simulink model "gm_parallel_delay_compensation_6phase"  (R2022a)
settings: Solver=FixedStepDiscrete  StartTime=0.0  StopTime=10.0  RelTol=1e-3
undefined symbols (not defined in the file or in its folder): f_c, L_d, L_q, L_x, L_y, p, psi_pm, R_ph
libraries: hdlmdlgenlib x10
settings Model: Creator=Andre Merx  LastModifiedBy=Andre Merx
settings SolverCC: AlgebraicLoopSolver=TrustRegion
settings DataIOCC: LimitDataPoints=on  SaveOutput=off  SaveTime=off
settings OptimizationCC: BlockReduction=off  ConditionallyExecuteInputs=off  DefaultParameterBehavior=Inlined  LifeSpan=inf
settings DebuggingCC: AlgebraicLoopMsg=error  InheritedTsInSrcMsg=none  SingleTaskRateTransMsg=error  UnconnectedInputMsg=warning  UnconnectedOutputMsg=warning  UnconnectedLineMsg=warning  AllowSymbolicDim=off  StrictBusMsg=ErrorOnBusTreatedAsVector  SFUnexpectedBacktrackingDiag=warning  SFNoUnconditionalDefaultTransitionDiag=warning  SFExecutionAtInitializationDiag=none  SFMachineParentedDataDiag=warning  ArithmeticOperatorsInVariantConditions=warning
settings HardwareCC: ProdBitPerPointer=32  ProdBitPerSizeT=32  ProdBitPerPtrDiffT=32  ProdLargestAtomicFloat=None  ProdIntDivRoundTo=Undefined  ProdEndianess=Unspecified  ProdWordSize=32  ProdHWDeviceType=ASIC/FPGA->ASIC/FPGA  ProdEqTarget=off
settings SFSimCC: SimUseLocalCustomCode=off  CustomCodeUndefinedFunction=UseInterfaceOnly
settings RTWCC: RTWUseLocalCustomCode=off
settings CodeAppCC: StateflowObjectComments=on
settings GRTTargetCC: TargetLangStandard=C89/C90 (ANSI)
settings ConfigComp: CovScope=ReferencedModels  CovMetricSettings=dw  CovSaveCumulativeToWorkspaceVar=on  CovSaveSingleToWorkspaceVar=on  CovExternalEMLEnable=off  CovSFcnEnable=off

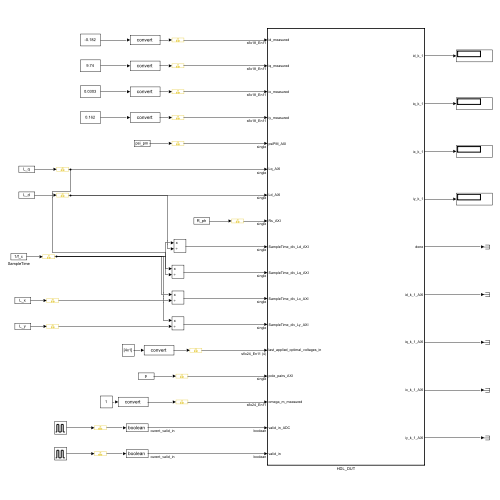
[thumbnail: Simulink's stored preview of the top-level diagram]
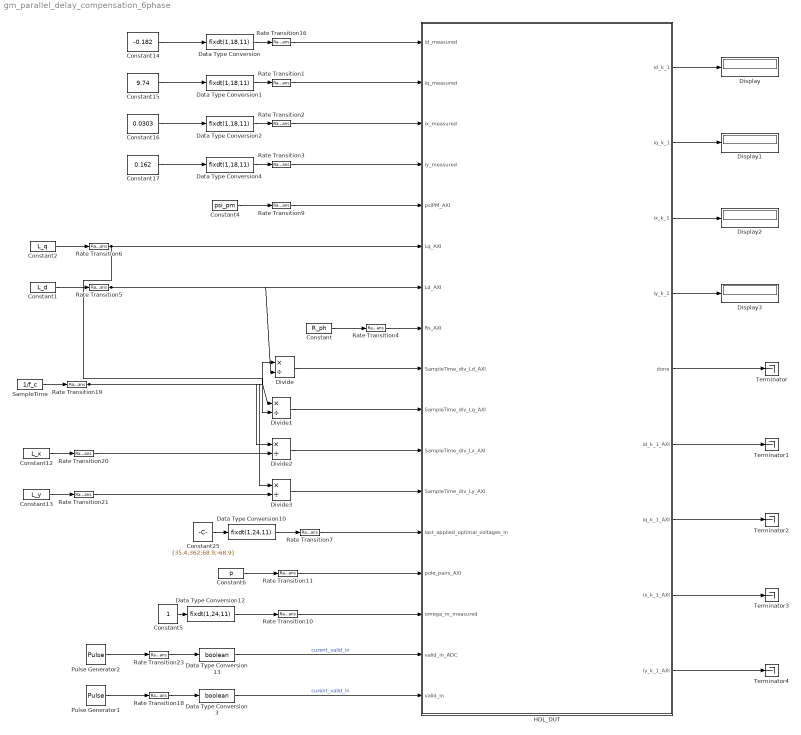
== system gm_parallel_delay_compensation_6phase ==
  Constant : Constant  Value=R_ph  OutDataTypeStr=single  SampleTime=-1
  Constant1 : Constant  Value=L_d  OutDataTypeStr=single  SampleTime=-1
  Constant12 : Constant  Value=L_x  OutDataTypeStr=single  SampleTime=-1
  Constant13 : Constant  Value=L_y  OutDataTypeStr=single  SampleTime=-1
  Constant14 : Constant  Value=-0.182
  Constant15 : Constant  Value=9.74
  Constant16 : Constant  Value=0.0303
  Constant17 : Constant  Value=0.162
  Constant2 : Constant  Value=L_q  OutDataTypeStr=single  SampleTime=-1
  Constant25 : Constant  Value=[35.4;362;68.9;-68.9]
  Constant4 : Constant  Value=psi_pm  OutDataTypeStr=single  SampleTime=-1
  Constant5 : Constant
  Constant6 : Constant  Value=p  OutDataTypeStr=single  SampleTime=-1
  Data Type Conversion{,1..2,4} (4 alike) : DataTypeConversion  OutDataTypeStr=fixdt(1,18,11)  SaturateOnIntegerOverflow=off  RndMeth=Floor
  Data Type Conversion10 : DataTypeConversion  OutDataTypeStr=fixdt(1,24,11)  SaturateOnIntegerOverflow=off  RndMeth=Floor
  Data Type Conversion12 : DataTypeConversion  OutDataTypeStr=fixdt(1,24,11)  SaturateOnIntegerOverflow=off  RndMeth=Floor
  Data Type Conversion13 : DataTypeConversion  OutDataTypeStr=boolean  SaturateOnIntegerOverflow=off  RndMeth=Floor
  Data Type Conversion3 : DataTypeConversion  OutDataTypeStr=boolean  SaturateOnIntegerOverflow=off  RndMeth=Floor
  Display{,1..3} (4 alike) : Display
  Divide{,1..3} (4 alike) : Product  Inputs=*/  RndMeth=Zero  SaturateOnIntegerOverflow=on
  HDL_DUT : Subsystem  TreatAsAtomicUnit=on
  Pulse Generator1 : DiscretePulseGenerator  PulseType=Time based  Period=1/f_c
  Pulse Generator2 : DiscretePulseGenerator  PulseType=Time based  Period=1/f_c
  Rate Transition{1..7,9..11,16,18..21,23} (16 alike) : RateTransition  OutPortSampleTime=Rt
  SampleTime : Constant  Value=1/f_c  OutDataTypeStr=single  SampleTime=-1
  Terminator{,1..4} (5 alike) : Terminator
  wires:
  Rate Transition7/1 -> HDL_DUT/13(last_applied_optimal_voltages_in)
  Data Type Conversion13/1 -> HDL_DUT/16(valid_in_ADC)  "curent_valid_in"
  Rate Transition23/1 -> Data Type Conversion13/1
  Pulse Generator2/1 -> Rate Transition23/1
  HDL_DUT/9(iy_k_1_AXI) -> Terminator4/1
  HDL_DUT/8(ix_k_1_AXI) -> Terminator3/1
  HDL_DUT/7(iq_k_1_AXI) -> Terminator2/1
  HDL_DUT/6(id_k_1_AXI) -> Terminator1/1
  Data Type Conversion10/1 -> Rate Transition7/1
  HDL_DUT/5(done) -> Terminator/1
  HDL_DUT/4(iy_k_1) -> Display3/1
  HDL_DUT/3(ix_k_1) -> Display2/1
  HDL_DUT/2(iq_k_1) -> Display1/1
  HDL_DUT/1(id_k_1) -> Display/1
  Constant17/1 -> Data Type Conversion4/1
  Rate Transition16/1 -> HDL_DUT/1(id_measured)
  Constant15/1 -> Data Type Conversion1/1
  Rate Transition1/1 -> HDL_DUT/2(iq_measured)
  Data Type Conversion4/1 -> Rate Transition3/1
  Rate Transition4/1 -> HDL_DUT/8(Rs_AXI)
  Rate Transition5/1 -> Divide/2, HDL_DUT/7(Ld_AXI)
  Constant6/1 -> Rate Transition11/1
  Constant16/1 -> Data Type Conversion2/1
  Data Type Conversion/1 -> Rate Transition16/1
  Constant4/1 -> Rate Transition9/1
  Data Type Conversion2/1 -> Rate Transition2/1
  Data Type Conversion1/1 -> Rate Transition1/1
  Constant14/1 -> Data Type Conversion/1
  Rate Transition3/1 -> HDL_DUT/4(iy_measured)
  Rate Transition2/1 -> HDL_DUT/3(ix_measured)
  Rate Transition10/1 -> HDL_DUT/15(omega_m_measured)
  Rate Transition9/1 -> HDL_DUT/5(psiPM_AXI)
  Constant5/1 -> Data Type Conversion12/1
  Data Type Conversion12/1 -> Rate Transition10/1
  Constant/1 -> Rate Transition4/1
  Rate Transition6/1 -> Divide1/2, HDL_DUT/6(Lq_AXI)
  Constant1/1 -> Rate Transition5/1
  Constant2/1 -> Rate Transition6/1
  Data Type Conversion3/1 -> HDL_DUT/17(valid_in)  "curent_valid_in"
  Pulse Generator1/1 -> Rate Transition18/1
  Constant12/1 -> Rate Transition20/1
  Constant13/1 -> Rate Transition21/1
  Rate Transition19/1 -> Divide2/1, Divide3/1, Divide1/1, Divide/1
  Divide1/1 -> HDL_DUT/10(SampleTime_div_Lq_AXI)
  Rate Transition11/1 -> HDL_DUT/14(pole_pairs_AXI)
  Rate Transition20/1 -> Divide2/2
  Divide3/1 -> HDL_DUT/12(SampleTime_div_Ly_AXI)
  Rate Transition18/1 -> Data Type Conversion3/1
  Rate Transition21/1 -> Divide3/2
  Divide2/1 -> HDL_DUT/11(SampleTime_div_Lx_AXI)
  SampleTime/1 -> Rate Transition19/1
  Divide/1 -> HDL_DUT/9(SampleTime_div_Ld_AXI)
  Constant25/1 -> Data Type Conversion10/1

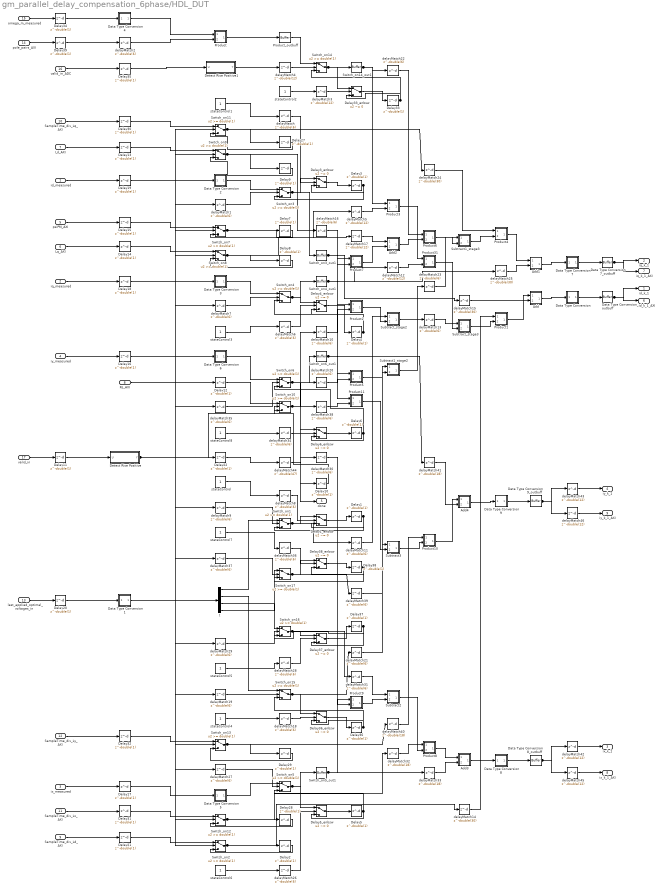
== system gm_parallel_delay_compensation_6phase/HDL_DUT ==
  id_measured : Inport  OutDataTypeStr=fixdt(1, 18, 11)  PortDimensions=1  SampleTime=1e-08
  iq_measured : Inport  Port=2  OutDataTypeStr=fixdt(1, 18, 11)  PortDimensions=1  SampleTime=1e-08
  ix_measured : Inport  Port=3  OutDataTypeStr=fixdt(1, 18, 11)  PortDimensions=1  SampleTime=1e-08
  iy_measured : Inport  Port=4  OutDataTypeStr=fixdt(1, 18, 11)  PortDimensions=1  SampleTime=1e-08
  psiPM_AXI : Inport  Port=5  OutDataTypeStr=single  PortDimensions=1  SampleTime=1e-08
  Lq_AXI : Inport  Port=6  OutDataTypeStr=single  PortDimensions=1  SampleTime=1e-08
  Ld_AXI : Inport  Port=7  OutDataTypeStr=single  PortDimensions=1  SampleTime=1e-08
  Rs_AXI : Inport  Port=8  OutDataTypeStr=single  PortDimensions=1  SampleTime=1e-08
  SampleTime_div_Ld_AXI : Inport  Port=9  OutDataTypeStr=single  PortDimensions=1  SampleTime=1e-08
  SampleTime_div_Lq_AXI : Inport  Port=10  OutDataTypeStr=single  PortDimensions=1  SampleTime=1e-08
  SampleTime_div_Lx_AXI : Inport  Port=11  OutDataTypeStr=single  PortDimensions=1  SampleTime=1e-08
  SampleTime_div_Ly_AXI : Inport  Port=12  OutDataTypeStr=single  PortDimensions=1  SampleTime=1e-08
  last_applied_optimal_voltages_in : Inport  Port=13  OutDataTypeStr=fixdt(1, 24, 11)  PortDimensions=[4]  SampleTime=1e-08
  pole_pairs_AXI : Inport  Port=14  OutDataTypeStr=single  PortDimensions=1  SampleTime=1e-08
  omega_m_measured : Inport  Port=15  OutDataTypeStr=fixdt(1, 24, 11)  PortDimensions=1  SampleTime=1e-08
  valid_in_ADC : Inport  Port=16  OutDataTypeStr=boolean  PortDimensions=1  SampleTime=1e-08
  valid_in : Inport  Port=17  OutDataTypeStr=boolean  PortDimensions=1  SampleTime=1e-08
  Add : Subsystem
      mask Display: disp('NFP\nadd');
  Add1 : Subsystem
      mask Display: disp('NFP\nadd');
  Add2 : Subsystem
      mask Display: disp('NFP\nadd');
  Add3 : Subsystem
      mask Display: disp('NFP\nadd');
  Add4 : Subsystem
      mask Display: disp('NFP\nadd');
  Data Type Conversion : Subsystem
      mask Display: disp('NFP\nconv');
  Data Type Conversion1 : Subsystem
      mask Display: disp('NFP\nconv');
  Data Type Conversion2 : Subsystem
      mask Display: disp('NFP\nconv');
  Data Type Conversion3 : Subsystem
      mask Display: disp('NFP\nconv');
  Data Type Conversion4 : Subsystem
      mask Display: disp('NFP\nconv');
  Data Type Conversion5 : Subsystem
      mask Display: disp('NFP\nconv');
  Data Type Conversion6 : Subsystem
      mask Display: disp('NFP\nconv');
  Data Type Conversion7 : Subsystem
      mask Display: disp('NFP\nconv');
  Data Type Conversion7_outbuff : hdlmdlgenlib/Buffer
      settings: SourceProductBaseCode=SL
  Data Type Conversion8 : Subsystem
      mask Display: disp('NFP\nconv');
  Data Type Conversion8_outbuff : hdlmdlgenlib/Buffer
      settings: SourceProductBaseCode=SL
  Data Type Conversion9 : Subsystem
      mask Display: disp('NFP\nconv');
  Data Type Conversion9_outbuff : hdlmdlgenlib/Buffer
      settings: SourceProductBaseCode=SL
  Data Type Conversion_outbuff : hdlmdlgenlib/Buffer
      settings: SourceProductBaseCode=SL
  Delay{1..22,27..39} (35 alike) : Delay  DelayLength=double(1)  InitialCondition=0  SampleTime=1e-08
  Delay1_enbsw : Switch  Criteria=u2 ~= 0  Threshold=double(0)  OutDataTypeStr=single  SampleTime=1e-08  SaturateOnIntegerOverflow=off  InputSameDT=off
  Delay33_enbsw : Switch  Criteria=u2 ~= 0  Threshold=double(0)  OutDataTypeStr=single  SampleTime=1e-08  SaturateOnIntegerOverflow=off  InputSameDT=off
  Delay36_enbsw : Switch  Criteria=u2 ~= 0  Threshold=double(0)  OutDataTypeStr=single  SampleTime=1e-08  SaturateOnIntegerOverflow=off  InputSameDT=off
  Delay37_enbsw : Switch  Criteria=u2 ~= 0  Threshold=double(0)  OutDataTypeStr=single  SampleTime=1e-08  SaturateOnIntegerOverflow=off  InputSameDT=off
  Delay38_enbsw : Switch  Criteria=u2 ~= 0  Threshold=double(0)  OutDataTypeStr=single  SampleTime=1e-08  SaturateOnIntegerOverflow=off  InputSameDT=off
  Delay3_enbsw : Switch  Criteria=u2 ~= 0  Threshold=double(0)  OutDataTypeStr=single  SampleTime=1e-08  SaturateOnIntegerOverflow=off  InputSameDT=off
  Delay4_enbsw : Switch  Criteria=u2 ~= 0  Threshold=double(0)  OutDataTypeStr=single  SampleTime=1e-08  SaturateOnIntegerOverflow=off  InputSameDT=off
  Delay5_enbsw : Switch  Criteria=u2 ~= 0  Threshold=double(0)  OutDataTypeStr=single  SampleTime=1e-08  SaturateOnIntegerOverflow=off  InputSameDT=off
  Delay6_enbsw : Switch  Criteria=u2 ~= 0  Threshold=double(0)  OutDataTypeStr=single  SampleTime=1e-08  SaturateOnIntegerOverflow=off  InputSameDT=off
  Detect Rise Positive : Subsystem  mask(Detect Rise Positive){vinit=double(0), InputProcessing=Elements as channels (sample based), OutDataTypeStr=boolean}
      mask prompts: vinit "Simulink:masks:InitialCondition_MP"; InputProcessing "Simulink:masks:InputProcessing_MP"; OutDataTypeStr "Simulink:masks:OutputDataType_MP"
      mask help: Simulink:masks:DetectRisePositive_MD
      mask init:
      | InputProcessing = 'Elements as channels (sample based)';
      | OutDataTypeStr = 'boolean';
      | vinit = double(0);
      mask TypeOptions InputProcessing: Simulink:masks:ColumnsAsChannelsFrameBased | Simulink:masks:ElementsAsChannelsSampleBased
      mask TypeOptions OutDataTypeStr: Simulink:masks:uint8 | Simulink:masks:boolean
      mask Display: fprintf('U > 0\n&  NOT\nU/z > 0')
  Detect Rise Positive1 : Subsystem  mask(Detect Rise Positive){vinit=double(0), InputProcessing=Elements as channels (sample based), OutDataTypeStr=boolean}
      mask prompts: vinit "Simulink:masks:InitialCondition_MP"; InputProcessing "Simulink:masks:InputProcessing_MP"; OutDataTypeStr "Simulink:masks:OutputDataType_MP"
      mask help: Simulink:masks:DetectRisePositive_MD
      mask init:
      | InputProcessing = 'Elements as channels (sample based)';
      | OutDataTypeStr = 'boolean';
      | vinit = double(0);
      mask TypeOptions InputProcessing: Simulink:masks:ColumnsAsChannelsFrameBased | Simulink:masks:ElementsAsChannelsSampleBased
      mask TypeOptions OutDataTypeStr: Simulink:masks:uint8 | Simulink:masks:boolean
      mask Display: fprintf('U > 0\n&  NOT\nU/z > 0')
  Product : Subsystem
      mask Display: disp('NFP\nmul');
  Product1 : Subsystem
      mask Display: disp('NFP\nmul');
  Product10 : Subsystem
      mask Display: disp('NFP\nmul');
  Product11 : Subsystem
      mask Display: disp('NFP\nmul');
  Product2 : Subsystem
      mask Display: disp('NFP\nmul');
  Product3 : Subsystem
      mask Display: disp('NFP\nmul');
  Product31 : Subsystem
      mask Display: disp('NFP\nmul');
  Product4 : Subsystem
      mask Display: disp('NFP\nmul');
  Product5 : Subsystem
      mask Display: disp('NFP\nmul');
  Product6 : Subsystem
      mask Display: disp('NFP\nmul');
  Product7 : Subsystem
      mask Display: disp('NFP\nmul');
  Product8 : Subsystem
      mask Display: disp('NFP\nmul');
  Product9 : Subsystem
      mask Display: disp('NFP\nmul');
  Product_outbuff : hdlmdlgenlib/Buffer
      settings: SourceProductBaseCode=SL
  Subtract1_stage2 : Subsystem
      mask Display: disp('NFP\nadd');
  Subtract1_stage3 : Subsystem
      mask Display: disp('NFP\nadd');
  Subtract2 : Subsystem
      mask Display: disp('NFP\nadd');
  Subtract3 : Subsystem
      mask Display: disp('NFP\nadd');
  Subtract_stage2 : Subsystem
      mask Display: disp('NFP\nadd');
  Subtract_stage3 : Subsystem
      mask Display: disp('NFP\nadd');
  Switch_on{1..17} (17 alike) : Switch  Threshold=double(1)  OutDataTypeStr=single  RndMeth=Simplest  SampleTime=1e-08  SaturateOnIntegerOverflow=off  InputSameDT=off
  Switch_on14_out1 : hdlmdlgenlib/Buffer
      settings: SourceProductBaseCode=SL
  Switch_on3_out1 : hdlmdlgenlib/Buffer
      settings: SourceProductBaseCode=SL
  Switch_on4_out1 : hdlmdlgenlib/Buffer
      settings: SourceProductBaseCode=SL
  Switch_on5_out1 : hdlmdlgenlib/Buffer
      settings: SourceProductBaseCode=SL
  Switch_on6_out1 : hdlmdlgenlib/Buffer
      settings: SourceProductBaseCode=SL
  delayMatch{,1..2,6..11,13,16,18..23,26..31,34..39} (29 alike) : Delay  DelayLength=double(6)  InitialCondition=0  SampleTime=1e-08
  delayMatch{3..5,12,17,42..43,45..46} (9 alike) : Delay  DelayLength=double(12)  InitialCondition=0  SampleTime=1e-08
  delayMatch{14..15,24..25} (4 alike) : Delay  DelayLength=double(30)  InitialCondition=0  SampleTime=1e-08
  delayMatch{32..33,40..41} (4 alike) : Delay  DelayLength=double(18)  InitialCondition=0  SampleTime=1e-08
  delayMatch44 : Delay  DelayLength=double(47)  InitialCondition=0  SampleTime=1e-08
  stateControl{,1..8} (9 alike) : Constant  OutDataTypeStr=boolean  SampleTime=1e-08
  t : Demux
  id_k_1 : Outport  SampleTime=1e-08
  iq_k_1 : Outport  Port=2  SampleTime=1e-08
  ix_k_1 : Outport  Port=3  SampleTime=1e-08
  iy_k_1 : Outport  Port=4  SampleTime=1e-08
  done : Outport  Port=5  SampleTime=1e-08
  id_k_1_AXI : Outport  Port=6  SampleTime=1e-08
  iq_k_1_AXI : Outport  Port=7  SampleTime=1e-08
  ix_k_1_AXI : Outport  Port=8  SampleTime=1e-08
  iy_k_1_AXI : Outport  Port=9  SampleTime=1e-08
  wires:
  id_measured/1 -> Delay19/1
  iq_measured/1 -> Delay18/1
  ix_measured/1 -> Delay17/1
  iy_measured/1 -> Delay16/1
  psiPM_AXI/1 -> Delay15/1
  Lq_AXI/1 -> Delay14/1
  Ld_AXI/1 -> Delay13/1
  Rs_AXI/1 -> Delay12/1
  SampleTime_div_Ld_AXI/1 -> Delay21/1
  SampleTime_div_Lq_AXI/1 -> Delay30/1
  SampleTime_div_Lx_AXI/1 -> Delay31/1
  SampleTime_div_Ly_AXI/1 -> Delay32/1
  last_applied_optimal_voltages_in/1 -> Delay20/1
  pole_pairs_AXI/1 -> Delay39/1
  omega_m_measured/1 -> Delay34/1
  valid_in_ADC/1 -> Delay35/1
  valid_in/1 -> Delay11/1
  Data Type Conversion_outbuff/1 -> id_k_1_AXI/1, id_k_1/1
  Data Type Conversion7_outbuff/1 -> iq_k_1_AXI/1, iq_k_1/1
  delayMatch42/1 -> ix_k_1/1
  delayMatch43/1 -> iy_k_1/1
  Delay11/1 -> Detect Rise Positive/1(U)
  Delay12/1 -> Switch_on10/1
  Delay13/1 -> Switch_on9/1
  Delay14/1 -> Switch_on8/1
  Delay15/1 -> Switch_on7/1
  Delay16/1 -> Data Type Conversion6/1(In1)
  Delay17/1 -> Data Type Conversion5/1(In1)
  Delay18/1 -> Data Type Conversion3/1(In1)
  Delay19/1 -> Data Type Conversion2/1(In1)
  Delay20/1 -> Data Type Conversion1/1(In1)
  Delay21/1 -> Switch_on2/1
  delayMatch44/1 -> done/1
  Delay30/1 -> Switch_on11/1
  Delay31/1 -> Switch_on12/1
  Delay32/1 -> Switch_on13/1
  Delay34/1 -> Data Type Conversion4/1(In1)
  Delay35/1 -> Detect Rise Positive1/1(U)
  delayMatch2/1 -> Product/2(In2)
  delayMatch1/1 -> Switch_on3/2
  delayMatch4/1 -> Switch_on14/2
  Product_outbuff/1 -> Switch_on14/1
  delayMatch11/1 -> Subtract_stage2/1(In1)
  delayMatch10/1 -> Product2/2(In2)
  delayMatch24/1 -> Product4/1(In1)
  delayMatch32/1 -> Product8/1(In1)
  delayMatch40/1 -> Product10/1(In1)
  delayMatch22/1 -> Product6/1(In1)
  delayMatch21/1 -> Subtract1_stage2/1(In1)
  delayMatch31/1 -> Subtract2/1(In1)
  delayMatch39/1 -> Subtract3/1(In1)
  delayMatch14/1 -> Product1/1(In1)
  delayMatch15/1 -> Add/2(In2)
  delayMatch12/1 -> Product31/2(In2)
  delayMatch33/1 -> Add3/2(In2)
  delayMatch41/1 -> Add4/2(In2)
  delayMatch17/1 -> Add2/1(In1)
  delayMatch5/1 -> Product3/2(In2)
  delayMatch16/1 -> Product7/2(In2)
  t/1 -> Switch_on1/1
  t/2 -> Switch_on15/1
  t/3 -> Switch_on16/1
  t/4 -> Switch_on17/1
  delayMatch13/1 -> Subtract_stage3/1(In1)
  delayMatch23/1 -> Subtract1_stage3/1(In1)
  Add/1(Out1) -> Data Type Conversion/1(In1)
  Add1/1(Out1) -> Data Type Conversion7/1(In1)
  Add2/1(Out1) -> Product6/2(In2)
  Add3/1(Out1) -> Data Type Conversion8/1(In1)
  Add4/1(Out1) -> Data Type Conversion9/1(In1)
  Data Type Conversion/1(Out1) -> Data Type Conversion_outbuff/1
  Data Type Conversion1/1(Out1) -> t/1
  Data Type Conversion2/1(Out1) -> Switch_on3/1
  Data Type Conversion3/1(Out1) -> Switch_on4/1
  Data Type Conversion4/1(Out1) -> Product/1(In1)
  Data Type Conversion5/1(Out1) -> Switch_on5/1
  Data Type Conversion6/1(Out1) -> Switch_on6/1
  Data Type Conversion7/1(Out1) -> Data Type Conversion7_outbuff/1
  Data Type Conversion8/1(Out1) -> Data Type Conversion8_outbuff/1
  Data Type Conversion9/1(Out1) -> Data Type Conversion9_outbuff/1
  Product/1(Out1) -> Product_outbuff/1
  Product1/1(Out1) -> Add/1(In1)
  Product10/1(Out1) -> Add4/1(In1)
  Product11/1(Out1) -> Subtract3/2(In2)
  Product2/1(Out1) -> Subtract_stage2/2(In2)
  Product3/1(Out1) -> Product31/1(In1)
  Product31/1(Out1) -> Subtract_stage3/2(In2)
  Product4/1(Out1) -> Add1/1(In1)
  Product5/1(Out1) -> Subtract1_stage2/2(In2)
  Product6/1(Out1) -> Subtract1_stage3/2(In2)
  Product7/1(Out1) -> Add2/2(In2)
  Product8/1(Out1) -> Add3/1(In1)
  Product9/1(Out1) -> Subtract2/2(In2)
  Subtract_stage2/1(Out1) -> delayMatch13/1
  Subtract_stage3/1(Out1) -> Product1/2(In2)
  Subtract1_stage2/1(Out1) -> delayMatch23/1
  Subtract1_stage3/1(Out1) -> Product4/2(In2)
  Subtract2/1(Out1) -> Product8/2(In2)
  Subtract3/1(Out1) -> Product10/2(In2)
  delayMatch8/1 -> Delay1_enbsw/2
  delayMatch/1 -> Delay3_enbsw/2
  delayMatch3/1 -> Delay33_enbsw/2
  delayMatch6/1 -> Delay4_enbsw/2
  delayMatch18/1 -> Delay36_enbsw/2
  delayMatch28/1 -> Delay37_enbsw/2
  delayMatch26/1 -> Delay5_enbsw/2
  delayMatch36/1 -> Delay38_enbsw/2
  delayMatch34/1 -> Delay6_enbsw/2
  stateControl1/1 -> delayMatch/1
  delayMatch7/1 -> Switch_on4/2
  Delay39/1 -> delayMatch2/1
  stateControl2/1 -> delayMatch3/1
  Detect Rise Positive1/1(Y) -> delayMatch4/1
  Switch_on8/1 -> delayMatch5/1, Delay8/1
  stateControl3/1 -> delayMatch6/1
  delayMatch9/1 -> Switch_on1/2
  stateControl/1 -> delayMatch8/1
  delayMatch19/1 -> Switch_on15/2
  delayMatch20/1 -> Product5/2(In2)
  delayMatch25/1 -> Add1/2(In2)
  Switch_on2/1 -> delayMatch14/1, Delay2/1
  Switch_on3_out1/1 -> delayMatch15/1, Product7/1(In1), Product2/1(In1)
  Switch_on9/1 -> delayMatch16/1, Delay9/1
  Switch_on7/1 -> delayMatch17/1, Delay7/1
  stateControl4/1 -> delayMatch18/1
  delayMatch27/1 -> Switch_on5/2
  delayMatch30/1 -> Product9/2(In2)
  Switch_on14_out1/1 -> delayMatch22/1, Product3/1(In1)
  Switch_on11/1 -> delayMatch24/1, Delay27/1
  Switch_on4_out1/1 -> delayMatch25/1, delayMatch12/1, Product5/1(In1)
  stateControl6/1 -> delayMatch26/1
  delayMatch29/1 -> Switch_on16/2
  stateControl5/1 -> delayMatch28/1
  delayMatch35/1 -> Switch_on6/2
  delayMatch38/1 -> Product11/2(In2)
  Switch_on12/1 -> delayMatch32/1, Delay28/1
  Switch_on5_out1/1 -> delayMatch33/1, Product9/1(In1)
  stateControl8/1 -> delayMatch34/1
  delayMatch37/1 -> Switch_on17/2
  stateControl7/1 -> delayMatch36/1
  Detect Rise Positive/1(Y) -> delayMatch37/1, delayMatch35/1, delayMatch29/1, delayMatch27/1, delayMatch19/1, delayMatch9/1, delayMatch7/1, delayMatch1/1, Delay22/1, Switch_on2/2, Switch_on10/2, Switch_on8/2, Switch_on11/2, Switch_on7/2, Switch_on9/2, Switch_on12/2, Switch_on13/2
  Switch_on10/1 -> delayMatch38/1, delayMatch30/1, delayMatch20/1, delayMatch10/1, Delay10/1
  Switch_on13/1 -> delayMatch40/1, Delay29/1
  Switch_on6_out1/1 -> delayMatch41/1, Product11/1(In1)
  delayMatch45/1 -> ix_k_1_AXI/1
  delayMatch46/1 -> iy_k_1_AXI/1
  Delay22/1 -> delayMatch44/1
  Data Type Conversion8_outbuff/1 -> delayMatch45/1, delayMatch42/1
  Data Type Conversion9_outbuff/1 -> delayMatch46/1, delayMatch43/1
  Switch_on1/1 -> delayMatch11/1, Delay1_enbsw/1
  Switch_on3/1 -> Switch_on3_out1/1, Delay3_enbsw/1
  Switch_on14/1 -> Switch_on14_out1/1, Delay33_enbsw/1
  Switch_on4/1 -> Switch_on4_out1/1, Delay4_enbsw/1
  Switch_on15/1 -> delayMatch21/1, Delay36_enbsw/1
  Switch_on16/1 -> delayMatch31/1, Delay37_enbsw/1
  Switch_on5/1 -> Switch_on5_out1/1, Delay5_enbsw/1
  Switch_on17/1 -> delayMatch39/1, Delay38_enbsw/1
  Switch_on6/1 -> Switch_on6_out1/1, Delay6_enbsw/1
  Delay2/1 -> Switch_on2/3
  Delay1_enbsw/1 -> Delay1/1
  Delay1/1 -> Switch_on1/3, Delay1_enbsw/3
  Delay3_enbsw/1 -> Delay3/1
  Delay3/1 -> Switch_on3/3, Delay3_enbsw/3
  Delay10/1 -> Switch_on10/3
  Delay33_enbsw/1 -> Delay33/1
  Delay33/1 -> Switch_on14/3, Delay33_enbsw/3
  Delay8/1 -> Switch_on8/3
  Delay4_enbsw/1 -> Delay4/1
  Delay4/1 -> Switch_on4/3, Delay4_enbsw/3
  Delay27/1 -> Switch_on11/3
  Delay36_enbsw/1 -> Delay36/1
  Delay36/1 -> Switch_on15/3, Delay36_enbsw/3
  Delay7/1 -> Switch_on7/3
  Delay9/1 -> Switch_on9/3
  Delay28/1 -> Switch_on12/3
  Delay37_enbsw/1 -> Delay37/1
  Delay37/1 -> Switch_on16/3, Delay37_enbsw/3
  Delay5_enbsw/1 -> Delay5/1
  Delay5/1 -> Switch_on5/3, Delay5_enbsw/3
  Delay29/1 -> Switch_on13/3
  Delay38_enbsw/1 -> Delay38/1
  Delay38/1 -> Switch_on17/3, Delay38_enbsw/3
  Delay6_enbsw/1 -> Delay6/1
  Delay6/1 -> Switch_on6/3, Delay6_enbsw/3

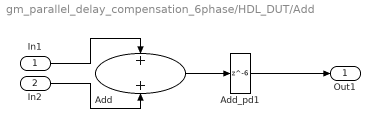
== system gm_parallel_delay_compensation_6phase/HDL_DUT/Add ==
  In1 : Inport
  In2 : Inport  Port=2
  Add : Sum  OutDataTypeStr=single  SampleTime=1e-08
  Add_pd1 : Delay  DelayLength=6
  Out1 : Outport
  wires:
  In1/1 -> Add/1
  In2/1 -> Add/2
  Add/1 -> Add_pd1/1
  Add_pd1/1 -> Out1/1

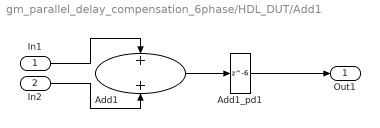
== system gm_parallel_delay_compensation_6phase/HDL_DUT/Add1 ==
  In1 : Inport
  In2 : Inport  Port=2
  Add1 : Sum  OutDataTypeStr=single  SampleTime=1e-08
  Add1_pd1 : Delay  DelayLength=6
  Out1 : Outport
  wires:
  In1/1 -> Add1/1
  In2/1 -> Add1/2
  Add1/1 -> Add1_pd1/1
  Add1_pd1/1 -> Out1/1

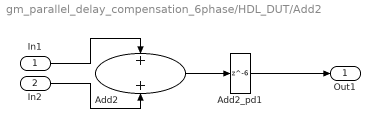
== system gm_parallel_delay_compensation_6phase/HDL_DUT/Add2 ==
  In1 : Inport
  In2 : Inport  Port=2
  Add2 : Sum  OutDataTypeStr=single  SampleTime=1e-08
  Add2_pd1 : Delay  DelayLength=6
  Out1 : Outport
  wires:
  In1/1 -> Add2/1
  In2/1 -> Add2/2
  Add2/1 -> Add2_pd1/1
  Add2_pd1/1 -> Out1/1

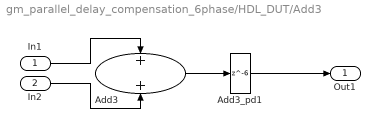
== system gm_parallel_delay_compensation_6phase/HDL_DUT/Add3 ==
  In1 : Inport
  In2 : Inport  Port=2
  Add3 : Sum  OutDataTypeStr=single  SampleTime=1e-08
  Add3_pd1 : Delay  DelayLength=6
  Out1 : Outport
  wires:
  In1/1 -> Add3/1
  In2/1 -> Add3/2
  Add3/1 -> Add3_pd1/1
  Add3_pd1/1 -> Out1/1

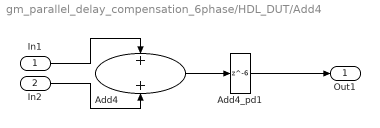
== system gm_parallel_delay_compensation_6phase/HDL_DUT/Add4 ==
  In1 : Inport
  In2 : Inport  Port=2
  Add4 : Sum  OutDataTypeStr=single  SampleTime=1e-08
  Add4_pd1 : Delay  DelayLength=6
  Out1 : Outport
  wires:
  In1/1 -> Add4/1
  In2/1 -> Add4/2
  Add4/1 -> Add4_pd1/1
  Add4_pd1/1 -> Out1/1

== system gm_parallel_delay_compensation_6phase/HDL_DUT/Data Type Conversion ==
  In1 : Inport
  Data Type Conversion : DataTypeConversion  OutDataTypeStr=fixdt(1, 18, 11)  SampleTime=1e-08  SaturateOnIntegerOverflow=off  RndMeth=Floor
  Data Type Conversion_pd1 : Delay  DelayLength=6
  Out1 : Outport
  wires:
  In1/1 -> Data Type Conversion/1
  Data Type Conversion/1 -> Data Type Conversion_pd1/1
  Data Type Conversion_pd1/1 -> Out1/1

== system gm_parallel_delay_compensation_6phase/HDL_DUT/Data Type Conversion1 ==
  In1 : Inport
  Data Type Conversion1 : DataTypeConversion  OutDataTypeStr=single  RndMeth=Nearest  SampleTime=1e-08  SaturateOnIntegerOverflow=off
  Data Type Conversion1_pd1 : Delay  DelayLength=6
  Out1 : Outport
  wires:
  In1/1 -> Data Type Conversion1/1
  Data Type Conversion1/1 -> Data Type Conversion1_pd1/1
  Data Type Conversion1_pd1/1 -> Out1/1

== system gm_parallel_delay_compensation_6phase/HDL_DUT/Data Type Conversion2 ==
  In1 : Inport
  Data Type Conversion2 : DataTypeConversion  OutDataTypeStr=single  RndMeth=Nearest  SampleTime=1e-08  SaturateOnIntegerOverflow=off
  Data Type Conversion2_pd1 : Delay  DelayLength=6
  Out1 : Outport
  wires:
  In1/1 -> Data Type Conversion2/1
  Data Type Conversion2/1 -> Data Type Conversion2_pd1/1
  Data Type Conversion2_pd1/1 -> Out1/1

== system gm_parallel_delay_compensation_6phase/HDL_DUT/Data Type Conversion3 ==
  In1 : Inport
  Data Type Conversion3 : DataTypeConversion  OutDataTypeStr=single  RndMeth=Nearest  SampleTime=1e-08  SaturateOnIntegerOverflow=off
  Data Type Conversion3_pd1 : Delay  DelayLength=6
  Out1 : Outport
  wires:
  In1/1 -> Data Type Conversion3/1
  Data Type Conversion3/1 -> Data Type Conversion3_pd1/1
  Data Type Conversion3_pd1/1 -> Out1/1

== system gm_parallel_delay_compensation_6phase/HDL_DUT/Data Type Conversion4 ==
  In1 : Inport
  Data Type Conversion4 : DataTypeConversion  OutDataTypeStr=single  RndMeth=Nearest  SampleTime=1e-08  SaturateOnIntegerOverflow=off
  Data Type Conversion4_pd1 : Delay  DelayLength=6
  Out1 : Outport
  wires:
  In1/1 -> Data Type Conversion4/1
  Data Type Conversion4/1 -> Data Type Conversion4_pd1/1
  Data Type Conversion4_pd1/1 -> Out1/1

== system gm_parallel_delay_compensation_6phase/HDL_DUT/Data Type Conversion5 ==
  In1 : Inport
  Data Type Conversion5 : DataTypeConversion  OutDataTypeStr=single  RndMeth=Nearest  SampleTime=1e-08  SaturateOnIntegerOverflow=off
  Data Type Conversion5_pd1 : Delay  DelayLength=6
  Out1 : Outport
  wires:
  In1/1 -> Data Type Conversion5/1
  Data Type Conversion5/1 -> Data Type Conversion5_pd1/1
  Data Type Conversion5_pd1/1 -> Out1/1

== system gm_parallel_delay_compensation_6phase/HDL_DUT/Data Type Conversion6 ==
  In1 : Inport
  Data Type Conversion6 : DataTypeConversion  OutDataTypeStr=single  RndMeth=Nearest  SampleTime=1e-08  SaturateOnIntegerOverflow=off
  Data Type Conversion6_pd1 : Delay  DelayLength=6
  Out1 : Outport
  wires:
  In1/1 -> Data Type Conversion6/1
  Data Type Conversion6/1 -> Data Type Conversion6_pd1/1
  Data Type Conversion6_pd1/1 -> Out1/1

== system gm_parallel_delay_compensation_6phase/HDL_DUT/Data Type Conversion7 ==
  In1 : Inport
  Data Type Conversion7 : DataTypeConversion  OutDataTypeStr=fixdt(1, 18, 11)  SampleTime=1e-08  SaturateOnIntegerOverflow=off  RndMeth=Floor
  Data Type Conversion7_pd1 : Delay  DelayLength=6
  Out1 : Outport
  wires:
  In1/1 -> Data Type Conversion7/1
  Data Type Conversion7/1 -> Data Type Conversion7_pd1/1
  Data Type Conversion7_pd1/1 -> Out1/1

== system gm_parallel_delay_compensation_6phase/HDL_DUT/Data Type Conversion8 ==
  In1 : Inport
  Data Type Conversion8 : DataTypeConversion  OutDataTypeStr=fixdt(1, 18, 11)  SampleTime=1e-08  SaturateOnIntegerOverflow=off  RndMeth=Floor
  Data Type Conversion8_pd1 : Delay  DelayLength=6
  Out1 : Outport
  wires:
  In1/1 -> Data Type Conversion8/1
  Data Type Conversion8/1 -> Data Type Conversion8_pd1/1
  Data Type Conversion8_pd1/1 -> Out1/1

== system gm_parallel_delay_compensation_6phase/HDL_DUT/Data Type Conversion9 ==
  In1 : Inport
  Data Type Conversion9 : DataTypeConversion  OutDataTypeStr=fixdt(1, 18, 11)  SampleTime=1e-08  SaturateOnIntegerOverflow=off  RndMeth=Floor
  Data Type Conversion9_pd1 : Delay  DelayLength=6
  Out1 : Outport
  wires:
  In1/1 -> Data Type Conversion9/1
  Data Type Conversion9/1 -> Data Type Conversion9_pd1/1
  Data Type Conversion9_pd1/1 -> Out1/1

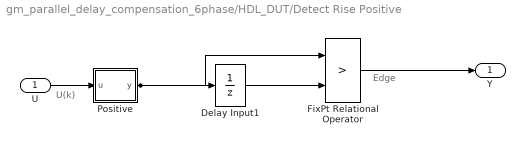
== system gm_parallel_delay_compensation_6phase/HDL_DUT/Detect Rise Positive ==
  note: Edge
  note: U(k)
  U : Inport  OutDataTypeStr=boolean  SampleTime=1e-08
  Delay Input1 : UnitDelay  Description=Store in Global RAM  DisableCoverage=on  InitialCondition=vinit  SampleTime=-1  HasFrameUpgradeWarning=on
  FixPt Relational Operator : RelationalOperator  Operator=>  OutDataTypeStr=boolean  ZeroCross=off  InputSameDT=off
  Positive : Subsystem  mask(Compare To Zero){relop=>, OutDataTypeStr=boolean, ZeroCross=off}
      mask prompts: relop "Simulink:masks:Operator_MP"; OutDataTypeStr "Simulink:masks:OutputDataType_MP"; ZeroCross "Simulink:masks:EnableZerocrossingDetection_MP"
      mask help: Simulink:masks:CompareToZero_MD
      mask init:
      | OutDataTypeStr = 'boolean';
      | ZeroCross = 'off';
      | blkName = 'parallel_delay_compensation_6phase/HDL_DUT/Detect Rise\nPositive/Positive';
      | relop = '>';
      | setValue = 'boolean';
      mask TypeOptions relop: == | ~= | < | <= | >= | >
      mask TypeOptions OutDataTypeStr: Simulink:masks:uint8 | Simulink:masks:boolean
      mask Callback ZeroCross: sl('zeroCrossEnable', gcbh);
      mask Display: disp([relop,' 0'])
  Y : Outport  SampleTime=1e-08
  wires:
  Delay Input1/1 -> FixPt Relational Operator/2
  FixPt Relational Operator/1 -> Y/1
  Positive/1(y) -> FixPt Relational Operator/1, Delay Input1/1
  U/1 -> Positive/1(u)

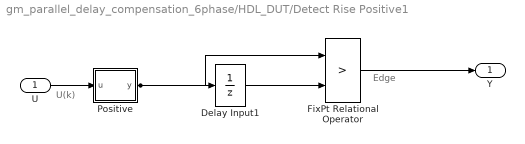
== system gm_parallel_delay_compensation_6phase/HDL_DUT/Detect Rise Positive1 ==
  note: Edge
  note: U(k)
  U : Inport  OutDataTypeStr=boolean  SampleTime=1e-08
  Delay Input1 : UnitDelay  Description=Store in Global RAM  DisableCoverage=on  InitialCondition=vinit  SampleTime=-1  HasFrameUpgradeWarning=on
  FixPt Relational Operator : RelationalOperator  Operator=>  OutDataTypeStr=boolean  ZeroCross=off  InputSameDT=off
  Positive : Subsystem  mask(Compare To Zero){relop=>, OutDataTypeStr=boolean, ZeroCross=off}
      mask prompts: relop "Simulink:masks:Operator_MP"; OutDataTypeStr "Simulink:masks:OutputDataType_MP"; ZeroCross "Simulink:masks:EnableZerocrossingDetection_MP"
      mask help: Simulink:masks:CompareToZero_MD
      mask init:
      | OutDataTypeStr = 'boolean';
      | ZeroCross = 'off';
      | blkName = 'parallel_delay_compensation_6phase/HDL_DUT/Detect Rise\nPositive1/Positive';
      | relop = '>';
      | setValue = 'boolean';
      mask TypeOptions relop: == | ~= | < | <= | >= | >
      mask TypeOptions OutDataTypeStr: Simulink:masks:uint8 | Simulink:masks:boolean
      mask Callback ZeroCross: sl('zeroCrossEnable', gcbh);
      mask Display: disp([relop,' 0'])
  Y : Outport  SampleTime=1e-08
  wires:
  Delay Input1/1 -> FixPt Relational Operator/2
  FixPt Relational Operator/1 -> Y/1
  Positive/1(y) -> FixPt Relational Operator/1, Delay Input1/1
  U/1 -> Positive/1(u)

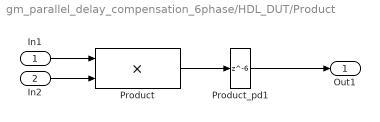
== system gm_parallel_delay_compensation_6phase/HDL_DUT/Product ==
  In1 : Inport
  In2 : Inport  Port=2
  Product : Product  Inputs=**  OutDataTypeStr=single  SampleTime=1e-08
  Product_pd1 : Delay  DelayLength=6
  Out1 : Outport
  wires:
  In1/1 -> Product/1
  In2/1 -> Product/2
  Product/1 -> Product_pd1/1
  Product_pd1/1 -> Out1/1

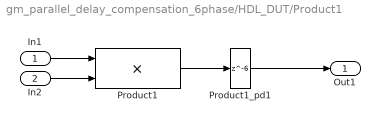
== system gm_parallel_delay_compensation_6phase/HDL_DUT/Product1 ==
  In1 : Inport
  In2 : Inport  Port=2
  Product1 : Product  Inputs=**  OutDataTypeStr=single  SampleTime=1e-08
  Product1_pd1 : Delay  DelayLength=6
  Out1 : Outport
  wires:
  In1/1 -> Product1/1
  In2/1 -> Product1/2
  Product1/1 -> Product1_pd1/1
  Product1_pd1/1 -> Out1/1

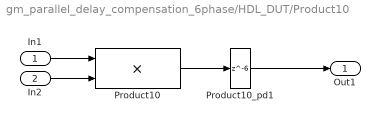
== system gm_parallel_delay_compensation_6phase/HDL_DUT/Product10 ==
  In1 : Inport
  In2 : Inport  Port=2
  Product10 : Product  Inputs=**  OutDataTypeStr=single  SampleTime=1e-08
  Product10_pd1 : Delay  DelayLength=6
  Out1 : Outport
  wires:
  In1/1 -> Product10/1
  In2/1 -> Product10/2
  Product10/1 -> Product10_pd1/1
  Product10_pd1/1 -> Out1/1

== system gm_parallel_delay_compensation_6phase/HDL_DUT/Product11 ==
  In1 : Inport
  In2 : Inport  Port=2
  Product11 : Product  Inputs=**  OutDataTypeStr=single  SampleTime=1e-08
  Product11_pd1 : Delay  DelayLength=6
  Out1 : Outport
  wires:
  In1/1 -> Product11/1
  In2/1 -> Product11/2
  Product11/1 -> Product11_pd1/1
  Product11_pd1/1 -> Out1/1

== system gm_parallel_delay_compensation_6phase/HDL_DUT/Product2 ==
  In1 : Inport
  In2 : Inport  Port=2
  Product2 : Product  Inputs=**  OutDataTypeStr=single  SampleTime=1e-08
  Product2_pd1 : Delay  DelayLength=6
  Out1 : Outport
  wires:
  In1/1 -> Product2/1
  In2/1 -> Product2/2
  Product2/1 -> Product2_pd1/1
  Product2_pd1/1 -> Out1/1

== system gm_parallel_delay_compensation_6phase/HDL_DUT/Product3 ==
  In1 : Inport
  In2 : Inport  Port=2
  Product3 : Product  Inputs=**  OutDataTypeStr=single  SampleTime=1e-08
  Product3_pd1 : Delay  DelayLength=6
  Out1 : Outport
  wires:
  In1/1 -> Product3/1
  In2/1 -> Product3/2
  Product3/1 -> Product3_pd1/1
  Product3_pd1/1 -> Out1/1

== system gm_parallel_delay_compensation_6phase/HDL_DUT/Product31 ==
  In1 : Inport
  In2 : Inport  Port=2
  Product31 : Product  Inputs=**  OutDataTypeStr=single  SampleTime=1e-08
  Product31_pd1 : Delay  DelayLength=6
  Out1 : Outport
  wires:
  In1/1 -> Product31/1
  In2/1 -> Product31/2
  Product31/1 -> Product31_pd1/1
  Product31_pd1/1 -> Out1/1

== system gm_parallel_delay_compensation_6phase/HDL_DUT/Product4 ==
  In1 : Inport
  In2 : Inport  Port=2
  Product4 : Product  Inputs=**  OutDataTypeStr=single  SampleTime=1e-08
  Product4_pd1 : Delay  DelayLength=6
  Out1 : Outport
  wires:
  In1/1 -> Product4/1
  In2/1 -> Product4/2
  Product4/1 -> Product4_pd1/1
  Product4_pd1/1 -> Out1/1

== system gm_parallel_delay_compensation_6phase/HDL_DUT/Product5 ==
  In1 : Inport
  In2 : Inport  Port=2
  Product5 : Product  Inputs=**  OutDataTypeStr=single  SampleTime=1e-08
  Product5_pd1 : Delay  DelayLength=6
  Out1 : Outport
  wires:
  In1/1 -> Product5/1
  In2/1 -> Product5/2
  Product5/1 -> Product5_pd1/1
  Product5_pd1/1 -> Out1/1

== system gm_parallel_delay_compensation_6phase/HDL_DUT/Product6 ==
  In1 : Inport
  In2 : Inport  Port=2
  Product6 : Product  Inputs=**  OutDataTypeStr=single  SampleTime=1e-08
  Product6_pd1 : Delay  DelayLength=6
  Out1 : Outport
  wires:
  In1/1 -> Product6/1
  In2/1 -> Product6/2
  Product6/1 -> Product6_pd1/1
  Product6_pd1/1 -> Out1/1

== system gm_parallel_delay_compensation_6phase/HDL_DUT/Product7 ==
  In1 : Inport
  In2 : Inport  Port=2
  Product7 : Product  Inputs=**  OutDataTypeStr=single  SampleTime=1e-08
  Product7_pd1 : Delay  DelayLength=6
  Out1 : Outport
  wires:
  In1/1 -> Product7/1
  In2/1 -> Product7/2
  Product7/1 -> Product7_pd1/1
  Product7_pd1/1 -> Out1/1

== system gm_parallel_delay_compensation_6phase/HDL_DUT/Product8 ==
  In1 : Inport
  In2 : Inport  Port=2
  Product8 : Product  Inputs=**  OutDataTypeStr=single  SampleTime=1e-08
  Product8_pd1 : Delay  DelayLength=6
  Out1 : Outport
  wires:
  In1/1 -> Product8/1
  In2/1 -> Product8/2
  Product8/1 -> Product8_pd1/1
  Product8_pd1/1 -> Out1/1

== system gm_parallel_delay_compensation_6phase/HDL_DUT/Product9 ==
  In1 : Inport
  In2 : Inport  Port=2
  Product9 : Product  Inputs=**  OutDataTypeStr=single  SampleTime=1e-08
  Product9_pd1 : Delay  DelayLength=6
  Out1 : Outport
  wires:
  In1/1 -> Product9/1
  In2/1 -> Product9/2
  Product9/1 -> Product9_pd1/1
  Product9_pd1/1 -> Out1/1

== system gm_parallel_delay_compensation_6phase/HDL_DUT/Subtract1_stage2 ==
  In1 : Inport
  In2 : Inport  Port=2
  Subtract1_stage2 : Sum  Inputs=+-  OutDataTypeStr=single  SampleTime=1e-08
  Subtract1_stage2_pd1 : Delay  DelayLength=6
  Out1 : Outport
  wires:
  In1/1 -> Subtract1_stage2/1
  In2/1 -> Subtract1_stage2/2
  Subtract1_stage2/1 -> Subtract1_stage2_pd1/1
  Subtract1_stage2_pd1/1 -> Out1/1

== system gm_parallel_delay_compensation_6phase/HDL_DUT/Subtract1_stage3 ==
  In1 : Inport
  In2 : Inport  Port=2
  Subtract1_stage3 : Sum  Inputs=+-  OutDataTypeStr=single  SampleTime=1e-08
  Subtract1_stage3_pd1 : Delay  DelayLength=6
  Out1 : Outport
  wires:
  In1/1 -> Subtract1_stage3/1
  In2/1 -> Subtract1_stage3/2
  Subtract1_stage3/1 -> Subtract1_stage3_pd1/1
  Subtract1_stage3_pd1/1 -> Out1/1

== system gm_parallel_delay_compensation_6phase/HDL_DUT/Subtract2 ==
  In1 : Inport
  In2 : Inport  Port=2
  Subtract2 : Sum  Inputs=+-  OutDataTypeStr=single  SampleTime=1e-08
  Subtract2_pd1 : Delay  DelayLength=6
  Out1 : Outport
  wires:
  In1/1 -> Subtract2/1
  In2/1 -> Subtract2/2
  Subtract2/1 -> Subtract2_pd1/1
  Subtract2_pd1/1 -> Out1/1

== system gm_parallel_delay_compensation_6phase/HDL_DUT/Subtract3 ==
  In1 : Inport
  In2 : Inport  Port=2
  Subtract3 : Sum  Inputs=+-  OutDataTypeStr=single  SampleTime=1e-08
  Subtract3_pd1 : Delay  DelayLength=6
  Out1 : Outport
  wires:
  In1/1 -> Subtract3/1
  In2/1 -> Subtract3/2
  Subtract3/1 -> Subtract3_pd1/1
  Subtract3_pd1/1 -> Out1/1

== system gm_parallel_delay_compensation_6phase/HDL_DUT/Subtract_stage2 ==
  In1 : Inport
  In2 : Inport  Port=2
  Subtract_stage2 : Sum  Inputs=+-  OutDataTypeStr=single  SampleTime=1e-08
  Subtract_stage2_pd1 : Delay  DelayLength=6
  Out1 : Outport
  wires:
  In1/1 -> Subtract_stage2/1
  In2/1 -> Subtract_stage2/2
  Subtract_stage2/1 -> Subtract_stage2_pd1/1
  Subtract_stage2_pd1/1 -> Out1/1

== system gm_parallel_delay_compensation_6phase/HDL_DUT/Subtract_stage3 ==
  In1 : Inport
  In2 : Inport  Port=2
  Subtract_stage3 : Sum  OutDataTypeStr=single  SampleTime=1e-08
  Subtract_stage3_pd1 : Delay  DelayLength=6
  Out1 : Outport
  wires:
  In1/1 -> Subtract_stage3/1
  In2/1 -> Subtract_stage3/2
  Subtract_stage3/1 -> Subtract_stage3_pd1/1
  Subtract_stage3_pd1/1 -> Out1/1

== system gm_parallel_delay_compensation_6phase/HDL_DUT/Detect Rise Positive/Positive ==
  u : Inport  OutDataTypeStr=boolean  SampleTime=1e-08
  Compare : RelationalOperator  Operator=>  OutDataTypeStr=boolean  ZeroCross=off
  Constant : Constant  DisableCoverage=on  Value=0  OutDataTypeStr=Inherit: Inherit via back propagation  SampleTime=-1  PreserveConstantTs=on
  y : Outport  SampleTime=1e-08
  wires:
  Compare/1 -> y/1
  Constant/1 -> Compare/2
  u/1 -> Compare/1

== system gm_parallel_delay_compensation_6phase/HDL_DUT/Detect Rise Positive1/Positive ==
  u : Inport  OutDataTypeStr=boolean  SampleTime=1e-08
  Compare : RelationalOperator  Operator=>  OutDataTypeStr=boolean  ZeroCross=off
  Constant : Constant  DisableCoverage=on  Value=0  OutDataTypeStr=Inherit: Inherit via back propagation  SampleTime=-1  PreserveConstantTs=on
  y : Outport  SampleTime=1e-08
  wires:
  Compare/1 -> y/1
  Constant/1 -> Compare/2
  u/1 -> Compare/1
